simulink model "modeloturbinadifg"  (R2022a)
settings: Solver=VariableStepAuto  StartTime=0.0  StopTime=1800  MaxStep=0.001  RelTol=1e-7
values from neighbouring files (symbols this model uses):
  Ag = 4    [parametrosturbina.m]
  alfa = 0.55    [parametrosturbina.m]
  alfai = 1.17    [parametrosturbina.m]
  altura = 85    [parametrosturbina.m]
  Ar = 4    [parametrosturbina.m]
  area = pi*radio^2    (= 3848.45100065)    [parametrosturbina.m]
  betaf = decay_factor*radio/v    (= 4.13636363636)    [parametrosturbina.m]
  betta = angulo_pala*pi/180    (= 0.0872664625997)    [parametrosturbina.m]
  Bt = 2836.49    [parametrosturbina.m]
  cuerda = 3    [parametrosturbina.m]
  densidad = 1.25    [parametrosturbina.m]
  dtotal = dbase+dtorre    (= 79920000)    [parametrosturbina.m]
  Itotal = Ibase+Itorre    (= 5108800000)    [parametrosturbina.m]
  Jt = 4.4535e5    (= 445350)    [parametrosturbina.m]
  K = Ls*Rr/Le    (= 5.9372867591)    [parametrosturbina.m]
  ktotal = kbase+ktorre    (= 3139900000)    [parametrosturbina.m]
  Le = Ls*Lr-Lm^2    (= 2.6996204624e-07)    [parametrosturbina.m]
  Lm = 1.526e-3    (= 0.001526)    [parametrosturbina.m]
  Ls = 1.61598e-3    (= 0.00161598)    [parametrosturbina.m]
  N = 83.5    [parametrosturbina.m]
  omega_s = 2*pi*60    (= 376.991118431)    [parametrosturbina.m]
  p = 2    [parametrosturbina.m]
  radio = 35    [parametrosturbina.m]
  Teg = 20    [parametrosturbina.m]
  Ter = 50    [parametrosturbina.m]
  thaui = 9    [parametrosturbina.m]
  Tsg = 10    [parametrosturbina.m]
  Tsr = 30    [parametrosturbina.m]
  v = 11    [parametrosturbina.m]
  Vs = 460*(2/3)^0.5    (= 375.588427227)    [parametrosturbina.m]
libraries: simulink x4
settings Model: Creator=afoa0  LastModifiedBy=afoa0
settings SolverCC: AlgebraicLoopSolver=TrustRegion
settings DebuggingCC: UnconnectedInputMsg=warning  UnconnectedOutputMsg=warning  UnconnectedLineMsg=warning  SFMachineParentedDataDiag=warning  UnderSpecifiedDimensionMsg=warning
settings RTWCC: DLArmComputeVersion=19.05

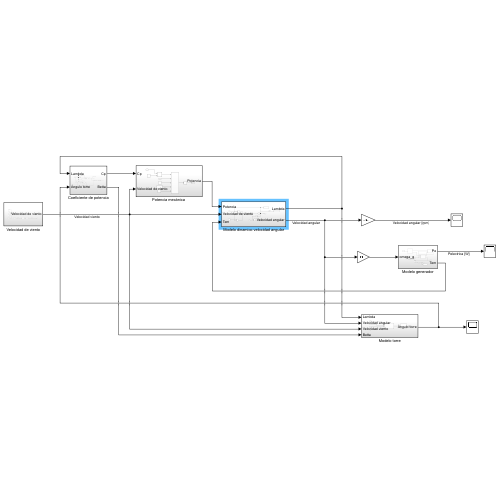
[thumbnail: Simulink's stored preview of the top-level diagram]
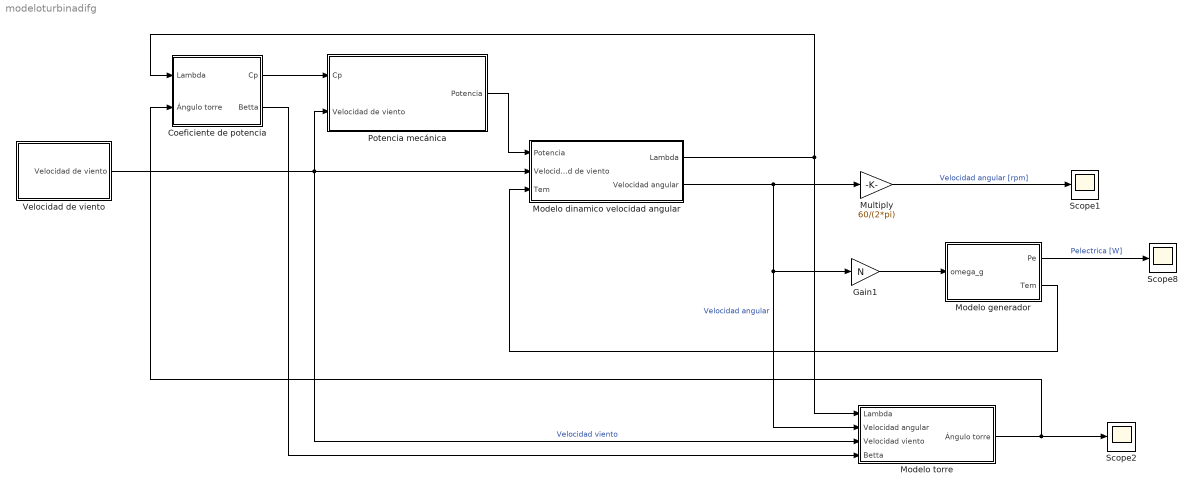
== system modeloturbinadifg ==
  Coeficiente de potencia : Subsystem
  Gain1 : Gain  Gain=N
  Modelo dinamico velocidad angular : Subsystem
  Modelo generador : Subsystem
  Modelo torre : Subsystem
  Multiply : Gain  Gain=60/(2*pi)
  "Potencia mecánica " : Subsystem
  Scope1 : Scope
  Scope2 : Scope
  Scope8 : Scope
  Velocidad de viento : Subsystem
  wires:
  Coeficiente de potencia/1(Cp) -> "Potencia mecánica "/1(Cp)
  "Potencia mecánica "/1(Potencia) -> Modelo dinamico velocidad angular/1(Potencia)
  Multiply/1 -> Scope1/1  "Velocidad angular [rpm]"
  Modelo generador/2(Tem) -> Modelo dinamico velocidad angular/3(Tem)
  Modelo generador/1(Pe) -> Scope8/1  "Pelectrica [W]"
  Gain1/1 -> Modelo generador/1(omega_g)
  Velocidad de viento/1(Velocidad de viento) -> Modelo torre/3(Velocidad viento), Modelo dinamico velocidad angular/2(Velocidad de viento), "Potencia mecánica "/2(Velocidad de viento)  "Velocidad viento"
  Modelo dinamico velocidad angular/2(Velocidad angular) -> Multiply/1, Modelo torre/2(Velocidad angular), Gain1/1  "Velocidad angular"
  Modelo dinamico velocidad angular/1(Lambda) -> Coeficiente de potencia/1(Lambda), Modelo torre/1(Lambda)
  Modelo torre/1(Ángulo torre) -> Coeficiente de potencia/2(Ángulo torre), Scope2/1
  Coeficiente de potencia/2(Betta) -> Modelo torre/4(Betta)

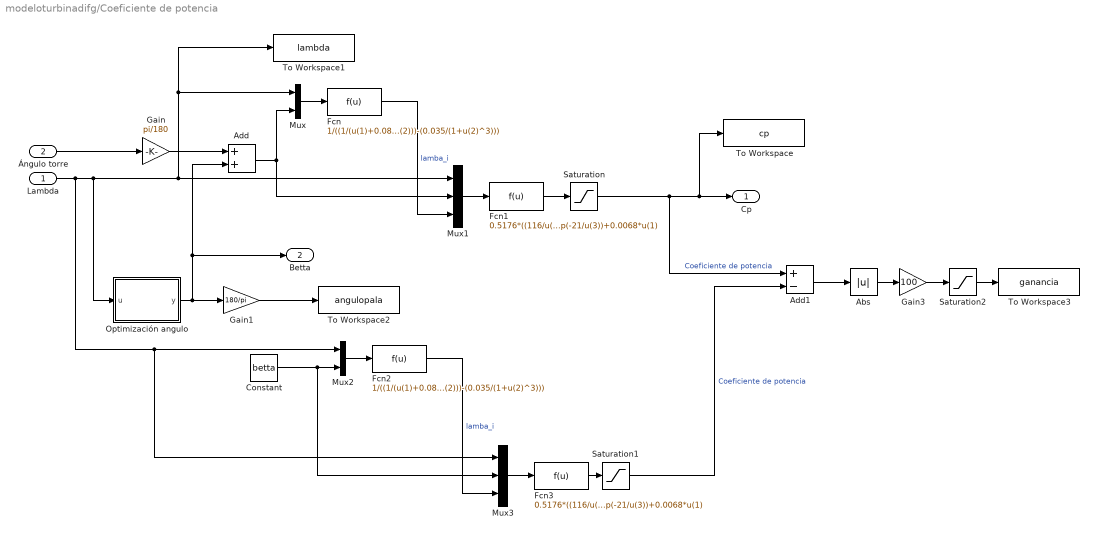
== system modeloturbinadifg/Coeficiente de potencia ==
  Lambda : Inport
  Ángulo torre : Inport  Port=2
  Abs : Abs  SaturateOnIntegerOverflow=off
  Add : Sum
  Add1 : Sum  Inputs=+-
  Constant : Constant  Value=betta
  Fcn : Fcn  Expr=1/((1/(u(1)+0.08*u(2)))-(0.035/(1+u(2)^3)))
  Fcn1 : Fcn  Expr=0.5176*((116/u(3))-0.4*u(2)-5)*exp(-21/u(3))+0.0068*u(1)
  Fcn2 : Fcn  Expr=1/((1/(u(1)+0.08*u(2)))-(0.035/(1+u(2)^3)))
  Fcn3 : Fcn  Expr=0.5176*((116/u(3))-0.4*u(2)-5)*exp(-21/u(3))+0.0068*u(1)
  Gain : Gain  Gain=pi/180
  Gain1 : Gain  Gain=180/pi
  Gain3 : Gain  Gain=100
  Mux : Mux  Inputs=2
  Mux1 : Mux  Inputs=3
  Mux2 : Mux  Inputs=2
  Mux3 : Mux  Inputs=3
  Optimización angulo : MATLAB Function  TreatAsAtomicUnit=on
  Saturation : Saturate  UpperLimit=0.6  LowerLimit=0
  Saturation1 : Saturate  UpperLimit=0.6  LowerLimit=0
  Saturation2 : Saturate  UpperLimit=0.3  LowerLimit=0
  To Workspace : ToWorkspace  VariableName=cp  SaveFormat=Timeseries  SampleTime=-1
  To Workspace1 : ToWorkspace  VariableName=lambda  SaveFormat=Timeseries  SampleTime=-1
  To Workspace2 : ToWorkspace  VariableName=angulopala  SaveFormat=Timeseries  SampleTime=-1
  To Workspace3 : ToWorkspace  VariableName=ganancia  SaveFormat=Timeseries  SampleTime=-1
  Cp : Outport
  Betta : Outport  Port=2
  wires:
  Mux/1 -> Fcn/1
  Fcn/1 -> Mux1/3  "lamba_i"
  Mux1/1 -> Fcn1/1
  Fcn1/1 -> Saturation/1
  Saturation/1 -> Add1/1, To Workspace/1, Cp/1  "Coeficiente de potencia"
  Gain1/1 -> To Workspace2/1
  Add/1 -> Mux1/2, Mux/2
  Ángulo torre/1 -> Gain/1
  Gain/1 -> Add/1
  Mux3/1 -> Fcn3/1
  Lambda/1 -> Mux3/1, Mux2/1, To Workspace1/1, Mux/1, Mux1/1, Optimización angulo/1(u)
  Fcn2/1 -> Mux3/3  "lamba_i"
  Saturation1/1 -> Add1/2  "Coeficiente de potencia"
  Mux2/1 -> Fcn2/1
  Fcn3/1 -> Saturation1/1
  Optimización angulo/1(y) -> Gain1/1, Betta/1, Add/2
  Add1/1 -> Abs/1
  Abs/1 -> Gain3/1
  Gain3/1 -> Saturation2/1
  Saturation2/1 -> To Workspace3/1
  Constant/1 -> Mux3/2, Mux2/2

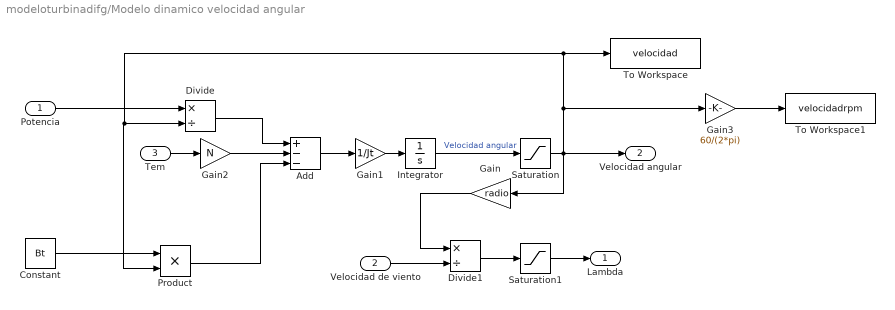
== system modeloturbinadifg/Modelo dinamico velocidad angular ==
  Potencia : Inport
  Velocidad de viento : Inport  Port=2
  Tem : Inport  Port=3
  Add : Sum  Inputs=+--
  Constant : Constant  Value=Bt
  Divide : Product  Inputs=*/
  Divide1 : Product  Inputs=*/
  Gain : Gain  Gain=radio
  Gain1 : Gain  Gain=1/Jt
  Gain2 : Gain  Gain=N
  Gain3 : Gain  Gain=60/(2*pi)
  Integrator : Integrator  InitialCondition=0.1
  Product : Product
  Saturation : Saturate  UpperLimit=6  LowerLimit=0.0001
  Saturation1 : Saturate  UpperLimit=30  LowerLimit=0
  To Workspace : ToWorkspace  VariableName=velocidad  SaveFormat=Timeseries  SampleTime=-1
  To Workspace1 : ToWorkspace  VariableName=velocidadrpm  SaveFormat=Timeseries  SampleTime=-1
  Lambda : Outport
  Velocidad angular : Outport  Port=2
  wires:
  Potencia/1 -> Divide/1
  Add/1 -> Gain1/1
  Gain1/1 -> Integrator/1
  Divide/1 -> Add/1
  Constant/1 -> Product/1
  Product/1 -> Add/3
  Gain/1 -> Divide1/1
  Velocidad de viento/1 -> Divide1/2
  Saturation/1 -> Gain/1, Velocidad angular/1, Product/2, Divide/2, To Workspace/1, Gain3/1
  Integrator/1 -> Saturation/1  "Velocidad angular"
  Tem/1 -> Gain2/1
  Gain2/1 -> Add/2
  Divide1/1 -> Saturation1/1
  Saturation1/1 -> Lambda/1
  Gain3/1 -> To Workspace1/1

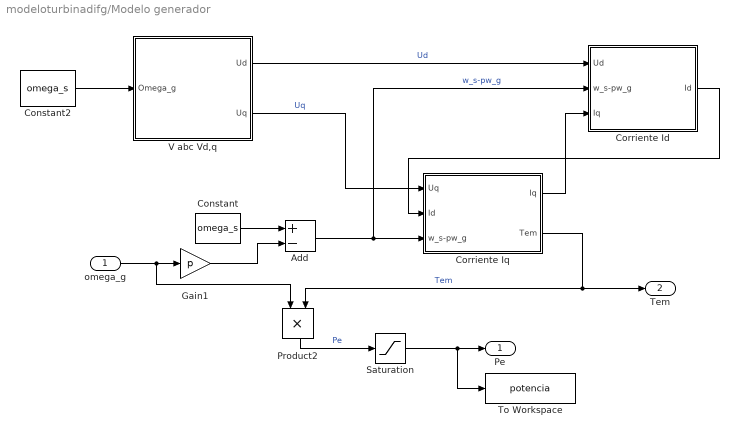
== system modeloturbinadifg/Modelo generador ==
  omega_g : Inport
  Add : Sum  Inputs=+-
  Constant : Constant  Value=omega_s
  Constant2 : Constant  Value=omega_s
  Corriente Id : Subsystem
  Corriente Iq : Subsystem
  Gain1 : Gain  Gain=p
  Product2 : Product
  Saturation : Saturate  UpperLimit=100e6  LowerLimit=0
  To Workspace : ToWorkspace  VariableName=potencia  SaveFormat=Timeseries  SampleTime=-1
  V abc Vd,q : Subsystem
  Pe : Outport
  Tem : Outport  Port=2
  wires:
  Corriente Iq/1(Iq) -> Corriente Id/3(Iq)
  omega_g/1 -> Gain1/1, Product2/1
  Constant2/1 -> V abc Vd,q/1(Omega_g)
  Gain1/1 -> Add/2
  Add/1 -> Corriente Id/2(w_s-pw_g), Corriente Iq/3(w_s-pw_g)  "w_s-pw_g"
  V abc Vd,q/1(Ud) -> Corriente Id/1(Ud)  "Ud"
  V abc Vd,q/2(Uq) -> Corriente Iq/1(Uq)  "Uq"
  Corriente Id/1(Id) -> Corriente Iq/2(Id)
  Corriente Iq/2(Tem) -> Product2/2, Tem/1  "Tem"
  Product2/1 -> Saturation/1  "Pe"
  Saturation/1 -> Pe/1, To Workspace/1
  Constant/1 -> Add/1

== system modeloturbinadifg/Modelo torre ==
  Lambda : Inport
  Velocidad angular : Inport  Port=2
  Velocidad viento : Inport  Port=3
  Betta : Inport  Port=4
  Cálculo de la fuerza aerodinámica : Subsystem
  Modelo segundo orden : Subsystem
  Ángulo torre : Outport
  wires:
  Lambda/1 -> Cálculo de la fuerza aerodinámica/1(Lambda)
  Velocidad viento/1 -> Cálculo de la fuerza aerodinámica/2(Velocidad viento)
  Velocidad angular/1 -> Cálculo de la fuerza aerodinámica/3(Velocidad angular)
  Betta/1 -> Cálculo de la fuerza aerodinámica/4(Betta)
  Cálculo de la fuerza aerodinámica/1(Pn) -> Modelo segundo orden/1(Pn)
  Modelo segundo orden/1(Ángulo Torre) -> Ángulo torre/1

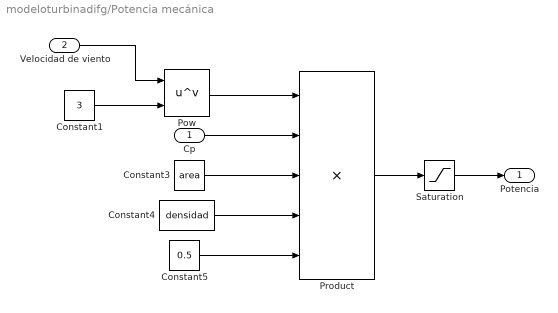
== system modeloturbinadifg/Potencia mecánica  ==
  Cp : Inport
  Velocidad de viento : Inport  Port=2
  Constant1 : Constant  Value=3
  Constant3 : Constant  Value=area
  Constant4 : Constant  Value=densidad
  Constant5 : Constant  Value=0.5
  Pow : Math  Operator=pow  SignedPower=on  RndMeth=Zero
  Product : Product  Inputs=5
  Saturation : Saturate  UpperLimit=10e6  LowerLimit=0
  Potencia : Outport
  wires:
  Constant3/1 -> Product/3
  Constant4/1 -> Product/4
  Constant5/1 -> Product/5
  Constant1/1 -> Pow/2
  Pow/1 -> Product/1
  Velocidad de viento/1 -> Pow/1
  Cp/1 -> Product/2
  Product/1 -> Saturation/1
  Saturation/1 -> Potencia/1

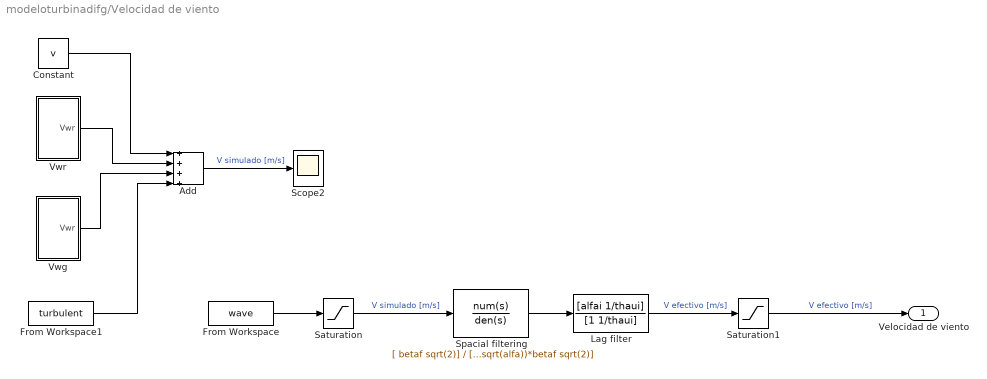
== system modeloturbinadifg/Velocidad de viento ==
  Add : Sum  Inputs=++++
  Constant : Constant  Value=v
  From Workspace : FromWorkspace  VariableName=wave  SampleTime=1  Interpolate=off  OutputAfterFinalValue=Setting to zero
  From Workspace1 : FromWorkspace  VariableName=turbulent  SampleTime=1  Interpolate=off  OutputAfterFinalValue=Setting to zero
  Lag filter : TransferFcn  Numerator=[alfai 1/thaui]  Denominator=[1 1/thaui]
  Saturation : Saturate  UpperLimit=50  LowerLimit=0
  Saturation1 : Saturate  UpperLimit=50  LowerLimit=0.0001
  Scope2 : Scope
  Spacial filtering : TransferFcn  Numerator=[ betaf sqrt(2)]  Denominator=[betaf^(2) (sqrt(2/alfa)+sqrt(alfa))*betaf sqrt(2)]
  Vwg : Subsystem
  Vwr : Subsystem
  Velocidad de viento : Outport
  wires:
  Vwr/1(Vwr) -> Add/2
  Constant/1 -> Add/1
  Vwg/1(Vwr) -> Add/3
  Add/1 -> Scope2/1  "V simulado [m/s]"
  Spacial filtering/1 -> Lag filter/1
  Lag filter/1 -> Saturation1/1  "V efectivo [m/s]"
  From Workspace/1 -> Saturation/1
  Saturation/1 -> Spacial filtering/1  "V simulado [m/s]"
  From Workspace1/1 -> Add/4
  Saturation1/1 -> Velocidad de viento/1  "V efectivo [m/s]"

== system modeloturbinadifg/Modelo generador/Corriente Id ==
  Ud : Inport
  w_s-pw_g : Inport  Port=2
  Iq : Inport  Port=3
  Add : Sum  Inputs=-++
  Gain : Gain  Gain=K
  Gain2 : Gain  Gain=Ls/Le
  Integrator : Integrator
  Product : Product
  Id : Outport
  wires:
  Product/1 -> Add/2
  Iq/1 -> Product/2
  Integrator/1 -> Gain/1, Id/1  "Id"
  Gain2/1 -> Add/3
  Gain/1 -> Add/1
  w_s-pw_g/1 -> Product/1
  Ud/1 -> Gain2/1
  Add/1 -> Integrator/1

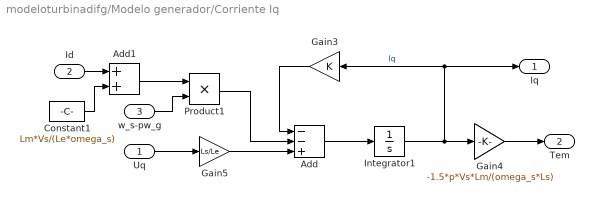
== system modeloturbinadifg/Modelo generador/Corriente Iq ==
  Uq : Inport
  Id : Inport  Port=2
  w_s-pw_g : Inport  Port=3
  Add : Sum  Inputs=--+
  Add1 : Sum
  Constant1 : Constant  Value=Lm*Vs/(Le*omega_s)
  Gain3 : Gain  Gain=K
  Gain4 : Gain  Gain=-1.5*p*Vs*Lm/(omega_s*Ls)
  Gain5 : Gain  Gain=Ls/Le
  Integrator1 : Integrator
  Product1 : Product
  Iq : Outport
  Tem : Outport  Port=2
  wires:
  Integrator1/1 -> Gain4/1, Gain3/1, Iq/1  "Iq"
  Product1/1 -> Add/2
  Constant1/1 -> Add1/2
  Id/1 -> Add1/1
  Uq/1 -> Gain5/1
  Gain5/1 -> Add/3
  Gain3/1 -> Add/1
  Gain4/1 -> Tem/1
  Add1/1 -> Product1/1
  w_s-pw_g/1 -> Product1/2
  Add/1 -> Integrator1/1

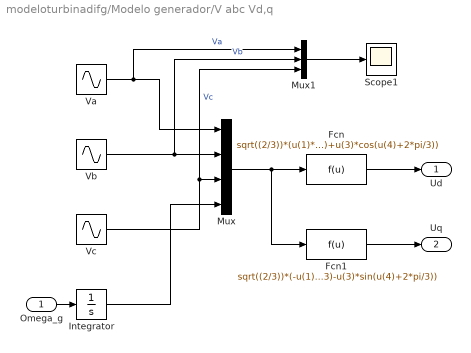
== system modeloturbinadifg/Modelo generador/V abc Vd,q ==
  Omega_g : Inport
  Fcn : Fcn  Expr=sqrt((2/3))*(u(1)*cos(u(4))+u(2)*cos(u(4)-2*pi/3)+u(3)*cos(u(4)+2*pi/3))
  Fcn1 : Fcn  Expr=sqrt((2/3))*(-u(1)*sin(u(4))-u(2)*sin(u(4)-2*pi/3)-u(3)*sin(u(4)+2*pi/3))
  Integrator : Integrator
  Mux : Mux
  Mux1 : Mux  Inputs=3
  Scope1 : Scope
  Va : Sin  Amplitude=Vs  Frequency=omega_s  SampleTime=0
  Vb : Sin  Amplitude=Vs  Frequency=omega_s  Phase=-2*pi/3  SampleTime=0
  Vc : Sin  Amplitude=Vs  Frequency=omega_s  Phase=2*pi/3  SampleTime=0
  Ud : Outport
  Uq : Outport  Port=2
  wires:
  Omega_g/1 -> Integrator/1
  Va/1 -> Mux1/1, Mux/1  "Va"
  Vb/1 -> Mux1/2, Mux/2  "Vb"
  Vc/1 -> Mux1/3, Mux/3  "Vc"
  Integrator/1 -> Mux/4
  Mux/1 -> Fcn1/1, Fcn/1
  Fcn/1 -> Ud/1
  Fcn1/1 -> Uq/1
  Mux1/1 -> Scope1/1

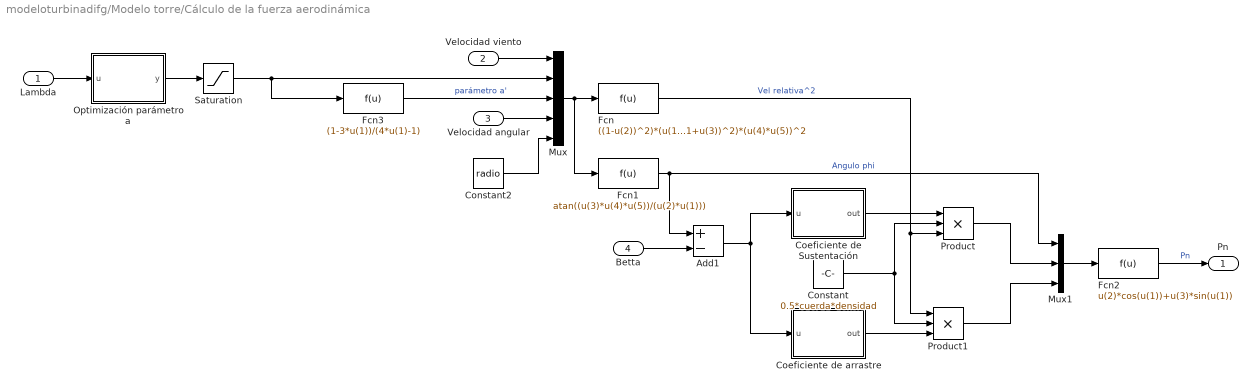
== system modeloturbinadifg/Modelo torre/Cálculo de la fuerza aerodinámica ==
  Lambda : Inport
  Velocidad viento : Inport  Port=2
  Velocidad angular : Inport  Port=3
  Betta : Inport  Port=4
  Add1 : Sum  Inputs=+-
  Coeficiente de Sustentación : MATLAB Function  TreatAsAtomicUnit=on
  Coeficiente de arrastre : MATLAB Function  TreatAsAtomicUnit=on
  Constant : Constant  Value=0.5*cuerda*densidad
  Constant2 : Constant  Value=radio
  Fcn : Fcn  Expr=((1-u(2))^2)*(u(1))^2+((1+u(3))^2)*(u(4)*u(5))^2
  Fcn1 : Fcn  Expr=atan((u(3)*u(4)*u(5))/(u(2)*u(1)))
  Fcn2 : Fcn  Expr=u(2)*cos(u(1))+u(3)*sin(u(1))
  Fcn3 : Fcn  Expr=(1-3*u(1))/(4*u(1)-1)
  Mux : Mux  Inputs=5
  Mux1 : Mux  Inputs=3
  Optimización parámetro a : MATLAB Function  TreatAsAtomicUnit=on
  Product : Product  Inputs=3
  Product1 : Product  Inputs=3
  Saturation : Saturate  UpperLimit=1  LowerLimit=0.001
  Pn : Outport
  wires:
  Saturation/1 -> Fcn3/1, Mux/2
  Fcn3/1 -> Mux/3  "parámetro a'"
  Fcn2/1 -> Pn/1  "Pn"
  Lambda/1 -> Optimización parámetro a/1(u)
  Coeficiente de Sustentación/1(out) -> Product/1
  Constant/1 -> Product1/2, Product/2
  Constant2/1 -> Mux/5
  Fcn1/1 -> Mux1/1, Add1/1  "Angulo phi"
  Fcn/1 -> Product1/1, Product/3  "Vel relativa^2"
  Mux/1 -> Fcn1/1, Fcn/1
  Mux1/1 -> Fcn2/1
  Optimización parámetro a/1(y) -> Saturation/1
  Add1/1 -> Coeficiente de arrastre/1(u), Coeficiente de Sustentación/1(u)
  Product/1 -> Mux1/2
  Velocidad angular/1 -> Mux/4
  Velocidad viento/1 -> Mux/1
  Product1/1 -> Mux1/3
  Coeficiente de arrastre/1(out) -> Product1/3
  Betta/1 -> Add1/2

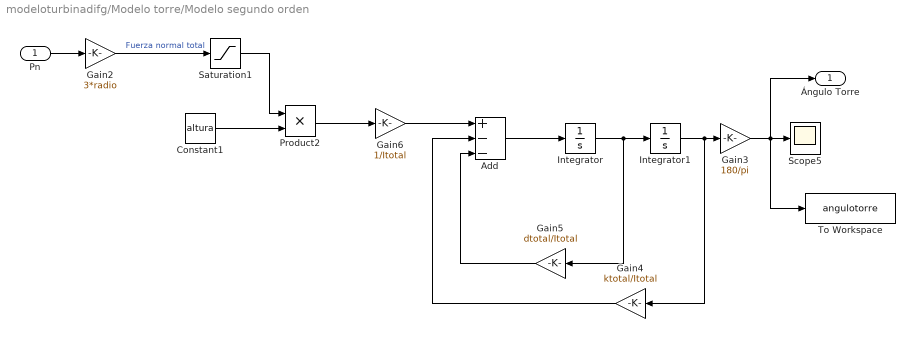
== system modeloturbinadifg/Modelo torre/Modelo segundo orden ==
  Pn : Inport
  Add : Sum  Inputs=+--
  Constant1 : Constant  Value=altura
  Gain2 : Gain  Gain=3*radio
  Gain3 : Gain  Gain=180/pi
  Gain4 : Gain  Gain=ktotal/Itotal
  Gain5 : Gain  Gain=dtotal/Itotal
  Gain6 : Gain  Gain=1/Itotal
  Integrator : Integrator
  Integrator1 : Integrator
  Product2 : Product
  Saturation1 : Saturate  UpperLimit=1e9  LowerLimit=0
  Scope5 : Scope
  To Workspace : ToWorkspace  VariableName=angulotorre  SaveFormat=Timeseries  SampleTime=-1
  Ángulo Torre : Outport
  wires:
  Integrator/1 -> Gain5/1, Integrator1/1
  Gain5/1 -> Add/3
  Integrator1/1 -> Gain4/1, Gain3/1
  Gain6/1 -> Add/1
  Constant1/1 -> Product2/2
  Product2/1 -> Gain6/1
  Gain2/1 -> Saturation1/1  "Fuerza normal total"
  Gain3/1 -> Ángulo Torre/1, To Workspace/1, Scope5/1
  Gain4/1 -> Add/2
  Add/1 -> Integrator/1
  Saturation1/1 -> Product2/1
  Pn/1 -> Gain2/1

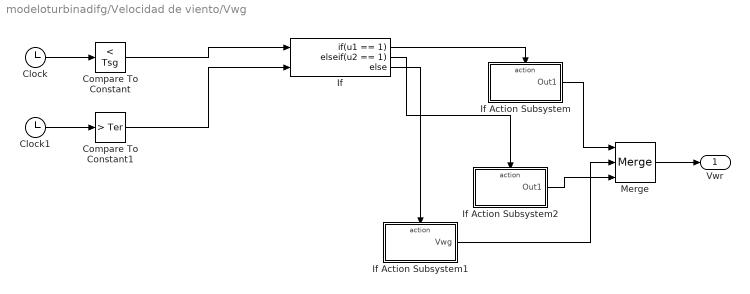
== system modeloturbinadifg/Velocidad de viento/Vwg ==
  Clock : Clock
  Clock1 : Clock
  Compare To Constant : simulink/Logic and Bit Operations/Compare To Constant  relop=<  const=Tsg  OutDataTypeStr=boolean
  Compare To Constant1 : simulink/Logic and Bit Operations/Compare To Constant  relop=>  const=Ter  OutDataTypeStr=boolean
  If : If  NumInputs=2  IfExpression=u1 == 1  ElseIfExpressions=u2 == 1
  If Action Subsystem : Subsystem  TreatAsAtomicUnit=on
  If Action Subsystem1 : Subsystem  TreatAsAtomicUnit=on
  If Action Subsystem2 : Subsystem  TreatAsAtomicUnit=on
  Merge : Merge  Inputs=3
  Vwr : Outport
  wires:
  If/1 -> If Action Subsystem/Action
  If Action Subsystem1/1(Vwg) -> Merge/2
  Compare To Constant/1 -> If/1
  If Action Subsystem/1(Out1) -> Merge/1
  Compare To Constant1/1 -> If/2
  If/3 -> If Action Subsystem1/Action
  If/2 -> If Action Subsystem2/Action
  Clock/1 -> Compare To Constant/1
  If Action Subsystem2/1(Out1) -> Merge/3
  Clock1/1 -> Compare To Constant1/1
  Merge/1 -> Vwr/1

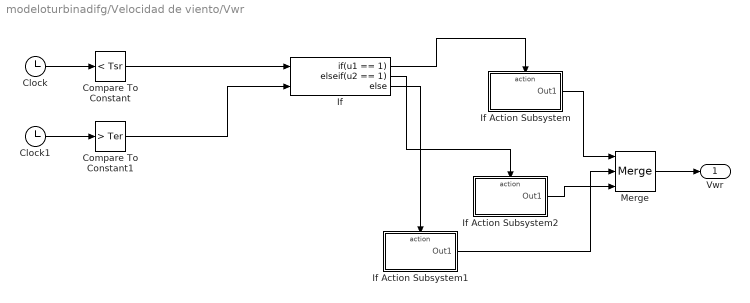
== system modeloturbinadifg/Velocidad de viento/Vwr ==
  Clock : Clock
  Clock1 : Clock
  Compare To Constant : simulink/Logic and Bit Operations/Compare To Constant  relop=<  const=Tsr  OutDataTypeStr=boolean
  Compare To Constant1 : simulink/Logic and Bit Operations/Compare To Constant  relop=>  const=Ter  OutDataTypeStr=boolean
  If : If  NumInputs=2  IfExpression=u1 == 1  ElseIfExpressions=u2 == 1
  If Action Subsystem : Subsystem  TreatAsAtomicUnit=on
  If Action Subsystem1 : Subsystem  TreatAsAtomicUnit=on
  If Action Subsystem2 : Subsystem  TreatAsAtomicUnit=on
  Merge : Merge  Inputs=3
  Vwr : Outport
  wires:
  If/1 -> If Action Subsystem/Action
  If Action Subsystem1/1(Out1) -> Merge/2
  Compare To Constant/1 -> If/1
  If Action Subsystem/1(Out1) -> Merge/1
  Compare To Constant1/1 -> If/2
  If/3 -> If Action Subsystem1/Action
  If/2 -> If Action Subsystem2/Action
  Clock/1 -> Compare To Constant/1
  If Action Subsystem2/1(Out1) -> Merge/3
  Clock1/1 -> Compare To Constant1/1
  Merge/1 -> Vwr/1

== system modeloturbinadifg/Velocidad de viento/Vwg/If Action Subsystem ==
  Action Port : ActionPort  ActionPortLabel=if(u1 == 1)
  Constant : Constant  Value=0
  Out1 : Outport
  wires:
  Constant/1 -> Out1/1

== system modeloturbinadifg/Velocidad de viento/Vwg/If Action Subsystem1 ==
  Action Port : ActionPort  ActionPortLabel=else
  Clock : Clock
  Fcn : Fcn  Expr=Ag*(1-cos(2*pi*((u(1)-Tsg)/Teg-Tsg)))
  Vwg : Outport
  wires:
  Fcn/1 -> Vwg/1
  Clock/1 -> Fcn/1

== system modeloturbinadifg/Velocidad de viento/Vwg/If Action Subsystem2 ==
  Action Port : ActionPort  ActionPortLabel=elseif(u2 == 1)
  Constant : Constant  Value=0
  Out1 : Outport
  wires:
  Constant/1 -> Out1/1

== system modeloturbinadifg/Velocidad de viento/Vwr/If Action Subsystem ==
  Action Port : ActionPort  ActionPortLabel=if(u1 == 1)
  Constant : Constant  Value=0
  Out1 : Outport
  wires:
  Constant/1 -> Out1/1

== system modeloturbinadifg/Velocidad de viento/Vwr/If Action Subsystem1 ==
  Action Port : ActionPort  ActionPortLabel=else
  Clock : Clock
  Constant : Constant  Value=Tsr
  Constant1 : Constant  Value=Ar
  Constant2 : Constant  Value=Ter-Tsr
  Divide : Product  Inputs=*/
  Product : Product
  Sum : Sum  Inputs=|-+
  Out1 : Outport
  wires:
  Constant/1 -> Sum/1
  Clock/1 -> Sum/2
  Sum/1 -> Product/2
  Constant1/1 -> Product/1
  Product/1 -> Divide/1
  Constant2/1 -> Divide/2
  Divide/1 -> Out1/1

== system modeloturbinadifg/Velocidad de viento/Vwr/If Action Subsystem2 ==
  Action Port : ActionPort  ActionPortLabel=elseif(u2 == 1)
  Constant : Constant  Value=Ar
  Out1 : Outport
  wires:
  Constant/1 -> Out1/1

== matlab function modeloturbinadifg/Modelo torre/Cálculo de la fuerza aerodinámica/Optimización parámetro a ==
  data: u input; y output [0..1]
function y = fcn(u)
raices=roots([16 -24 9-3*u^2 -1+u^2]);
r=real(raices);
m=find(r>=0 & r<=1);
z=r(m);
y = z(1);

== matlab function modeloturbinadifg/Modelo torre/Cálculo de la fuerza aerodinámica/Coeficiente de Sustentación ==
  data: u input; out output
function out = fcn(u)
if(u<-0.17453293)
    y=-1;
elseif (u>=-0.17453293 && u<=0.15707963)
y=7.0228*u+0.359;
else
    y=1.25;
end
out= y;

== matlab function modeloturbinadifg/Modelo torre/Cálculo de la fuerza aerodinámica/Coeficiente de arrastre ==
  data: u input; out output
function out = fcn(u)
if(u<-0.261799)
    y=2.5;
elseif (u>=-0.261799 && u<=0.261799)
y=13.661*u^4-0.2481*u^3-0.0108*u^2+0.0054*u+0.0077;
else
    y=2.5;
end

out=y;

== matlab function modeloturbinadifg/Coeficiente de potencia/Optimización angulo ==
  data: u input; y output
function y = fcn(u)
Cp=@(betta)-(0.5176*(116/(1/((1/(u+0.08*betta))-(0.035/(betta^3+1))))-0.4*betta-5)*exp(-21/(1/((1/(u+0.08*betta))-(0.035/(betta^3+1)))))+0.0068*u);

[x1,x2]=fminbnd(Cp,0,pi/2);

betta=x1;
Cp=-x2; % gives xmax=0.5959, ymax=0.2718
angulo=180*betta/pi;
y=betta;
